simulink model "FOC_Motor_Control"  (R2020b)
settings: Solver=FixedStepAuto  StartTime=0.0  StopTime=10.0  FixedStep=Fixed_Step_Size  RelTol=1e-3
values from neighbouring files (symbols this model uses):
  Angle = 1.0    [Hall_FOC_Data.sldd]
  Angle_offset = 0.1985    [Hall_FOC_Data.sldd]
  atan_table = -1.5690511 -1.5690503 -1.5690495 -1.5690485 -1.5690477 -1.5690469 -1.569046 -1.5690452 -1.5690442 -1.5690434 -1.5690426 -1.5690417 -1.5690409 -1.5690399 -1.5690391 -1.5690383 -1.5690374 -1.5690365 -1.5690356 -1.5690348 -1.5690339 -1.569033 -1.5690322 -1.5690314 -1.5690304 -1.5690296 -1.5690287 -1.5690278 -1.5690269 -1.5690261 -1.5690252 -1.5690243 -1.5690234 -1.5690225 -1.5690217 -1.5690207 -1.569    [Hall_FOC_Data.sldd]
  Cosine_table = 1.0 0.99999529 0.99999058 0.99998587 0.99998116 0.99996704 0.99995291 0.99993885 0.99992472 0.99990118 0.99987763 0.99985409 0.9998306 0.99979764 0.99976468 0.99973178 0.99969882 0.99965644 0.99961412 0.99957174 0.99952942 0.99947762 0.99942589 0.99937415 0.99932235 0.9992612 0.99920005 0.99913889 0.99907768 0.99900717 0.99893659 0.99886602 0.99879545 0.99871546 0.99863547 0.99855554 0.99847555 0.    [Hall_FOC_Data.sldd]
  Dead_Com_Enable = 0.0    [Hall_FOC_Data.sldd]
  Dead_Time = 0.0    [Hall_FOC_Data.sldd]
  FF_Enable = 0.0    [Hall_FOC_Data.sldd]
  Flux = 0.0260812    [Hall_FOC_Data.sldd]
  FluxWeak_Enable = 0.0    [Hall_FOC_Data.sldd]
  FluxWeak_Idref_max = 0.0    [Hall_FOC_Data.sldd]
  FluxWeak_Idref_min = -200.0    [Hall_FOC_Data.sldd]
  FluxWeak_Ki = 50.0    [Hall_FOC_Data.sldd]
  FluxWeak_Kp = 1.2    [Hall_FOC_Data.sldd]
  HaLL_AngleShift = -0.25    [Hall_FOC_Data.sldd]
  HaLL_Sector1 = 5.236    [Hall_FOC_Data.sldd]
  HaLL_Sector2 = 1.0472    [Hall_FOC_Data.sldd]
  HaLL_Sector3 = 0.0    [Hall_FOC_Data.sldd]
  HaLL_Sector4 = 3.1415    [Hall_FOC_Data.sldd]
  HaLL_Sector5 = 4.1888    [Hall_FOC_Data.sldd]
  HaLL_Sector6 = 2.0944    [Hall_FOC_Data.sldd]
  HaLL_Timer_T = 1.0E-5    [Hall_FOC_Data.sldd]
  Harmonic_Com_Enable = 0.0    [Hall_FOC_Data.sldd]
  Harmonic_Id5th_Ki = 32.0    [Hall_FOC_Data.sldd]
  Harmonic_Id5th_Kp = 1.2    [Hall_FOC_Data.sldd]
  Harmonic_Id5th_Max = 60.0    [Hall_FOC_Data.sldd]
  Harmonic_Id5th_Min = -60.0    [Hall_FOC_Data.sldd]
  Harmonic_Id7th_Ki = 24.0    [Hall_FOC_Data.sldd]
  Harmonic_Id7th_Kp = 0.8    [Hall_FOC_Data.sldd]
  Harmonic_Id7th_Max = 60.0    [Hall_FOC_Data.sldd]
  Harmonic_Id7th_Min = -60.0    [Hall_FOC_Data.sldd]
  Harmonic_Iq5th_Ki = 32.0    [Hall_FOC_Data.sldd]
  Harmonic_Iq5th_Kp = 1.2    [Hall_FOC_Data.sldd]
  Harmonic_Iq5th_Max = 60.0    [Hall_FOC_Data.sldd]
  Harmonic_Iq5th_Min = -60.0    [Hall_FOC_Data.sldd]
  Harmonic_Iq7th_Ki = 24.0    [Hall_FOC_Data.sldd]
  Harmonic_Iq7th_Kp = 0.8    [Hall_FOC_Data.sldd]
  Harmonic_Iq7th_Max = 60.0    [Hall_FOC_Data.sldd]
  Harmonic_Iq7th_Min = -60.0    [Hall_FOC_Data.sldd]
  ID_Ki = 0.8    [Hall_FOC_Data.sldd]
  ID_Kp = 3.2    [Hall_FOC_Data.sldd]
  IQ_Ki = 0.32    [Hall_FOC_Data.sldd]
  IQ_Kp = 3.3    [Hall_FOC_Data.sldd]
  LADRC_b0 = 80000.0    [Hall_FOC_Data.sldd]
  LADRC_Omega_c = 80.0    [Hall_FOC_Data.sldd]
  Ld = 0.004    [Hall_FOC_Data.sldd]
  Lq = 0.0042    [Hall_FOC_Data.sldd]
  MTPA_id_table = 0.22889 0.23462678 0.23770036 0.2381243 0.23591207 0.23107713 0.2236329 0.21359272 0.20096992 0.18577772 0.16802935 0.14773798 0.12491672 0.099578641 0.071736768 0.041404068 0.0085934745 -0.026682133 -0.064409919 -0.10457709 -0.14717092 -0.1921787 -0.2395878 -0.28938559 -0.34155953 -0.39609709 -0.45298585 -0.51221335 -0.57376724 -0.63763517 -0.70380485 -0.77226412 -0.84300071 -0.91600245 -0.991257    [Hall_FOC_Data.sldd]
  MTPA_iq_table = -1.0417 -0.16083497 0.71926296 1.5985928 2.4771533 3.3549435 4.2319627 5.1082091 5.9836826 6.8583813 7.732305 8.6054525 9.4778223 10.349415 11.220228 12.090261 12.959513 13.827983 14.69567 15.562573 16.428694 17.294027 18.158575 19.022335 19.885307 20.747492 21.608887 22.469492 23.329306 24.188328 25.046556 25.903992 26.760633 27.616482 28.471533 29.325788 30.179247 31.031908 31.883772 32.734837 3    [Hall_FOC_Data.sldd]
  MTPA_Te_Max = 800.0    [Hall_FOC_Data.sldd]
  MTPA_Te_Min = 0.0    [Hall_FOC_Data.sldd]
  Over_modulation = 0.0    [Hall_FOC_Data.sldd]
  Pole_Pairs = 2.0    [Hall_FOC_Data.sldd]
  PWM_Frequency = 10000.0    [Hall_FOC_Data.sldd]
  R = 0.4    [Hall_FOC_Data.sldd]
  Sine_table = 0.0 0.0015339879 0.0030679768 0.0046019657 0.0061359555 0.0076698866 0.0092038177 0.010737749 0.012271681 0.013805497 0.015339312 0.016873131 0.018406944 0.019940587 0.021474229 0.023007872 0.024541514 0.026074925 0.027608337 0.029141748 0.03067516 0.032208283 0.033741407 0.035274528 0.036807653 0.038340431 0.039873205 0.04140598 0.042938754 0.04447113 0.046003502 0.047535874 0.049068246 0.0506001    [Hall_FOC_Data.sldd]
  Speed_Ki = 0.633    [Hall_FOC_Data.sldd]
  Speed_Kp = 0.0267    [Hall_FOC_Data.sldd]
  Speed_PI_OutputMax = 5.0    [Hall_FOC_Data.sldd]
  Speed_PI_OutputMin = -5.0    [Hall_FOC_Data.sldd]
  SpeedFilter_Fn = 0.2    [Hall_FOC_Data.sldd]
  TorqueMode = 0.0    [Hall_FOC_Data.sldd]
undefined symbols (not defined in the file or in its folder): DiscIntNeverNeededParam, inverter, magnitude, SVPWM
libraries: simulink x6, powerlib_extras x4, pid_lib x1
(part 5 of 5)

== system FOC_Motor_Control/Motor_Control/Motor_Control_Function/FOC_Control_100us/FOC/DT_Compensation/DT_Compensation/Subsystem/Subsystem2 ==
  Voltage : Inport
  Action Port : ActionPort  ActionPortLabel=elseif((u1 >1.570796)&(u1<=2.617993))
  Gain : Gain  Gain=-1
  Gain1 : Gain
  Gain2 : Gain  Gain=-1
  Mux1 : Mux  Inputs=3
  Out1 : Outport
  wires:
  Mux1/1 -> Out1/1
  Voltage/1 -> Gain2/1, Gain1/1, Gain/1
  Gain/1 -> Mux1/1
  Gain1/1 -> Mux1/2
  Gain2/1 -> Mux1/3

== system FOC_Motor_Control/Motor_Control/Motor_Control_Function/FOC_Control_100us/FOC/DT_Compensation/DT_Compensation/Subsystem/Subsystem3 ==
  Voltage : Inport
  Action Port : ActionPort  ActionPortLabel=elseif((u1 >2.617993)&(u1<=3.665191))
  Gain : Gain  Gain=-1
  Gain1 : Gain
  Gain2 : Gain
  Mux1 : Mux  Inputs=3
  Out1 : Outport
  wires:
  Mux1/1 -> Out1/1
  Voltage/1 -> Gain2/1, Gain1/1, Gain/1
  Gain/1 -> Mux1/1
  Gain1/1 -> Mux1/2
  Gain2/1 -> Mux1/3

== system FOC_Motor_Control/Motor_Control/Motor_Control_Function/FOC_Control_100us/FOC/DT_Compensation/DT_Compensation/Subsystem/Subsystem4 ==
  Voltage : Inport
  Action Port : ActionPort  ActionPortLabel=elseif((u1 >3.665191)&(u1<=4.7123889))
  Gain : Gain  Gain=-1
  Gain1 : Gain  Gain=-1
  Gain2 : Gain
  Mux1 : Mux  Inputs=3
  Out1 : Outport
  wires:
  Mux1/1 -> Out1/1
  Voltage/1 -> Gain2/1, Gain1/1, Gain/1
  Gain/1 -> Mux1/1
  Gain1/1 -> Mux1/2
  Gain2/1 -> Mux1/3

== system FOC_Motor_Control/Motor_Control/Motor_Control_Function/FOC_Control_100us/FOC/DT_Compensation/DT_Compensation/Subsystem/Subsystem5 ==
  Voltage : Inport
  Action Port : ActionPort  ActionPortLabel=elseif((u1 >4.7123889)&(u1<=5.75958))
  Gain : Gain
  Gain1 : Gain  Gain=-1
  Gain2 : Gain
  Mux1 : Mux  Inputs=3
  Out1 : Outport
  wires:
  Mux1/1 -> Out1/1
  Voltage/1 -> Gain2/1, Gain1/1, Gain/1
  Gain/1 -> Mux1/1
  Gain1/1 -> Mux1/2
  Gain2/1 -> Mux1/3

== system FOC_Motor_Control/Motor_Control/Motor_Control_Function/FOC_Control_100us/FOC/Har_Compensation/Har_Compensation/Idq5/LPF ==
  u : Inport
  Add : Sum  Inputs=+-
  Add1 : Sum
  Constant1 : Constant  Value=0.005  OutDataTypeStr=single
  Divide1 : Product  Inputs=**
  Unit Delay : UnitDelay  SampleTime=-1  HasFrameUpgradeWarning=on
  y : Outport
  wires:
  Constant1/1 -> Divide1/1
  u/1 -> Add/1
  Add/1 -> Divide1/2
  Divide1/1 -> Add1/1
  Unit Delay/1 -> Add/2, Add1/2
  Add1/1 -> Unit Delay/1, y/1

== system FOC_Motor_Control/Motor_Control/Motor_Control_Function/FOC_Control_100us/FOC/Har_Compensation/Har_Compensation/Idq5/LPF2 ==
  u : Inport
  Add : Sum  Inputs=+-
  Add1 : Sum
  Constant1 : Constant  Value=0.005  OutDataTypeStr=single
  Divide1 : Product  Inputs=**
  Unit Delay : UnitDelay  SampleTime=-1  HasFrameUpgradeWarning=on
  y : Outport
  wires:
  Constant1/1 -> Divide1/1
  u/1 -> Add/1
  Add/1 -> Divide1/2
  Divide1/1 -> Add1/1
  Unit Delay/1 -> Add/2, Add1/2
  Add1/1 -> Unit Delay/1, y/1

== system FOC_Motor_Control/Motor_Control/Motor_Control_Function/FOC_Control_100us/FOC/Har_Compensation/Har_Compensation/Idq5/Park1 ==
  Ialf : Inport
  Ibelt : Inport  Port=2
  Cos_theta : Inport  Port=3
  Sin_theta : Inport  Port=4
  Fcn2 : Fcn  Expr=u(1)*u(3)+u(2)*u(4)
  Fcn3 : Fcn  Expr=u(2)*u(3)-u(1)*u(4)
  Mux : Mux
  Id5 : Outport  VectorParamsAs1DForOutWhenUnconnected=off
  Iq5 : Outport  Port=2  VectorParamsAs1DForOutWhenUnconnected=off
  wires:
  Fcn3/1 -> Iq5/1
  Fcn2/1 -> Id5/1
  Mux/1 -> Fcn3/1, Fcn2/1
  Sin_theta/1 -> Mux/4
  Cos_theta/1 -> Mux/3
  Ibelt/1 -> Mux/2
  Ialf/1 -> Mux/1

== system FOC_Motor_Control/Motor_Control/Motor_Control_Function/FOC_Control_100us/FOC/Har_Compensation/Har_Compensation/Idq7/LPF ==
  u : Inport
  Add : Sum  Inputs=+-
  Add1 : Sum
  Constant1 : Constant  Value=0.005  OutDataTypeStr=single
  Divide1 : Product  Inputs=**
  Unit Delay : UnitDelay  SampleTime=-1  HasFrameUpgradeWarning=on
  y : Outport
  wires:
  Constant1/1 -> Divide1/1
  u/1 -> Add/1
  Add/1 -> Divide1/2
  Divide1/1 -> Add1/1
  Unit Delay/1 -> Add/2, Add1/2
  Add1/1 -> Unit Delay/1, y/1

== system FOC_Motor_Control/Motor_Control/Motor_Control_Function/FOC_Control_100us/FOC/Har_Compensation/Har_Compensation/Idq7/LPF2 ==
  u : Inport
  Add : Sum  Inputs=+-
  Add1 : Sum
  Constant1 : Constant  Value=0.005  OutDataTypeStr=single
  Divide1 : Product  Inputs=**
  Unit Delay : UnitDelay  SampleTime=-1  HasFrameUpgradeWarning=on
  y : Outport
  wires:
  Constant1/1 -> Divide1/1
  u/1 -> Add/1
  Add/1 -> Divide1/2
  Divide1/1 -> Add1/1
  Unit Delay/1 -> Add/2, Add1/2
  Add1/1 -> Unit Delay/1, y/1

== system FOC_Motor_Control/Motor_Control/Motor_Control_Function/FOC_Control_100us/FOC/Har_Compensation/Har_Compensation/Idq7/Park1 ==
  Ialf : Inport
  Ibelt : Inport  Port=2
  Cos_theta : Inport  Port=3
  Sin_theta : Inport  Port=4
  Fcn2 : Fcn  Expr=u(1)*u(3)+u(2)*u(4)
  Fcn3 : Fcn  Expr=u(2)*u(3)-u(1)*u(4)
  Mux : Mux
  Id7 : Outport  VectorParamsAs1DForOutWhenUnconnected=off
  Iq7 : Outport  Port=2  VectorParamsAs1DForOutWhenUnconnected=off
  wires:
  Ialf/1 -> Mux/1
  Ibelt/1 -> Mux/2
  Cos_theta/1 -> Mux/3
  Sin_theta/1 -> Mux/4
  Mux/1 -> Fcn2/1, Fcn3/1
  Fcn2/1 -> Id7/1
  Fcn3/1 -> Iq7/1

== system FOC_Motor_Control/Motor_Control/Motor_Control_Function/FOC_Control_100us/FOC/Har_Compensation/Har_Compensation/idq57_Controller/I-park ==
  Ud5 : Inport
  Uq5 : Inport  Port=2
  Cos_theta : Inport  Port=3
  Sin_theta : Inport  Port=4
  Fcn : Fcn  Expr=u(1)*u(3)-u(2)*u(4)
  Fcn1 : Fcn  Expr=u(1)*u(4)+u(2)*u(3)
  Mux1 : Mux
  Ualfa5 : Outport  VectorParamsAs1DForOutWhenUnconnected=off
  Ubelt5 : Outport  Port=2  VectorParamsAs1DForOutWhenUnconnected=off
  wires:
  Uq5/1 -> Mux1/2
  Ud5/1 -> Mux1/1
  Fcn1/1 -> Ubelt5/1
  Fcn/1 -> Ualfa5/1
  Mux1/1 -> Fcn1/1, Fcn/1
  Sin_theta/1 -> Mux1/4
  Cos_theta/1 -> Mux1/3

== system FOC_Motor_Control/Motor_Control/Motor_Control_Function/FOC_Control_100us/FOC/Har_Compensation/Har_Compensation/idq57_Controller/I-park1 ==
  Ud7 : Inport
  Uq7 : Inport  Port=2
  Cos_theta : Inport  Port=3
  Sin_theta : Inport  Port=4
  Fcn : Fcn  Expr=u(1)*u(3)-u(2)*u(4)
  Fcn1 : Fcn  Expr=u(1)*u(4)+u(2)*u(3)
  Mux1 : Mux
  Ualfa7 : Outport  VectorParamsAs1DForOutWhenUnconnected=off
  Ubelt7 : Outport  Port=2  VectorParamsAs1DForOutWhenUnconnected=off
  wires:
  Ud7/1 -> Mux1/1
  Fcn/1 -> Ualfa7/1
  Mux1/1 -> Fcn1/1, Fcn/1
  Fcn1/1 -> Ubelt7/1
  Uq7/1 -> Mux1/2
  Cos_theta/1 -> Mux1/3
  Sin_theta/1 -> Mux1/4

== system FOC_Motor_Control/Motor_Control/Motor_Control_Function/FOC_Control_100us/FOC/Har_Compensation/Har_Compensation/idq57_Controller/ID_5 ==
  Err : Inport
  Add : Sum
  Discrete-Time Integrator : DiscreteIntegrator  SampleTime=-1  ICPrevOutput=DiscIntNeverNeededParam  ICPrevScaledInput=DiscIntNeverNeededParam
  Ki : Constant  Value=Harmonic_Id5th_Ki  OutDataTypeStr=single
  Kp : Constant  Value=Harmonic_Id5th_Kp  OutDataTypeStr=single
  Product : Product
  Product1 : Product
  Saturation : Saturate  UpperLimit=Harmonic_Id5th_Max  LowerLimit=Harmonic_Id5th_Min
  PI_Out : Outport
  wires:
  Kp/1 -> Product/1
  Err/1 -> Product1/2, Product/2
  Product1/1 -> Discrete-Time Integrator/1
  Product/1 -> Add/1
  Add/1 -> Saturation/1
  Saturation/1 -> PI_Out/1
  Discrete-Time Integrator/1 -> Add/2
  Ki/1 -> Product1/1

== system FOC_Motor_Control/Motor_Control/Motor_Control_Function/FOC_Control_100us/FOC/Har_Compensation/Har_Compensation/idq57_Controller/ID_7 ==
  Err : Inport
  Add : Sum
  Discrete-Time Integrator : DiscreteIntegrator  SampleTime=-1  ICPrevOutput=DiscIntNeverNeededParam  ICPrevScaledInput=DiscIntNeverNeededParam
  Ki : Constant  Value=Harmonic_Id7th_Ki  OutDataTypeStr=single
  Kp : Constant  Value=Harmonic_Id7th_Kp  OutDataTypeStr=single
  Product : Product
  Product1 : Product
  Saturation : Saturate  UpperLimit=Harmonic_Id7th_Max  LowerLimit=Harmonic_Id7th_Min
  PI_Out : Outport
  wires:
  Kp/1 -> Product/1
  Err/1 -> Product1/2, Product/2
  Product1/1 -> Discrete-Time Integrator/1
  Product/1 -> Add/1
  Add/1 -> Saturation/1
  Saturation/1 -> PI_Out/1
  Discrete-Time Integrator/1 -> Add/2
  Ki/1 -> Product1/1

== system FOC_Motor_Control/Motor_Control/Motor_Control_Function/FOC_Control_100us/FOC/Har_Compensation/Har_Compensation/idq57_Controller/IQ_5 ==
  Err : Inport
  Add : Sum
  Discrete-Time Integrator : DiscreteIntegrator  SampleTime=-1  ICPrevOutput=DiscIntNeverNeededParam  ICPrevScaledInput=DiscIntNeverNeededParam
  Ki : Constant  Value=Harmonic_Iq5th_Ki  OutDataTypeStr=single
  Kp : Constant  Value=Harmonic_Iq5th_Kp  OutDataTypeStr=single
  Product : Product
  Product1 : Product
  Saturation : Saturate  UpperLimit=Harmonic_Iq5th_Max  LowerLimit=Harmonic_Iq5th_Min
  PI_Out : Outport
  wires:
  Kp/1 -> Product/1
  Err/1 -> Product1/2, Product/2
  Product1/1 -> Discrete-Time Integrator/1
  Product/1 -> Add/1
  Add/1 -> Saturation/1
  Saturation/1 -> PI_Out/1
  Discrete-Time Integrator/1 -> Add/2
  Ki/1 -> Product1/1

== system FOC_Motor_Control/Motor_Control/Motor_Control_Function/FOC_Control_100us/FOC/Har_Compensation/Har_Compensation/idq57_Controller/IQ_7 ==
  Err : Inport
  Add : Sum
  Discrete-Time Integrator : DiscreteIntegrator  SampleTime=-1  ICPrevOutput=DiscIntNeverNeededParam  ICPrevScaledInput=DiscIntNeverNeededParam
  Ki : Constant  Value=Harmonic_Iq7th_Ki  OutDataTypeStr=single
  Kp : Constant  Value=Harmonic_Iq7th_Kp  OutDataTypeStr=single
  Product : Product
  Product1 : Product
  Saturation : Saturate  UpperLimit=Harmonic_Iq7th_Max  LowerLimit=Harmonic_Iq7th_Min
  PI_Out : Outport
  wires:
  Kp/1 -> Product/1
  Err/1 -> Product1/2, Product/2
  Product1/1 -> Discrete-Time Integrator/1
  Product/1 -> Add/1
  Add/1 -> Saturation/1
  Saturation/1 -> PI_Out/1
  Discrete-Time Integrator/1 -> Add/2
  Ki/1 -> Product1/1

== system FOC_Motor_Control/Motor_Control/Motor_Control_Function/FOC_Control_100us/FOC/Har_Compensation/Har_Compensation/idq57_Controller/Subsystem1 ==
  note: id
  note: we
  Id7 : Inport
  We : Inport  Port=2
  Iq7 : Inport  Port=3
  Fcn : Fcn  Expr=-u(2)*Lq*u(3)+R*u(1)
  Fcn1 : Fcn  Expr=u(2)*Ld*u(1)+R*u(3)
  Mux1 : Mux  Inputs=3
  Udc7 : Outport  VectorParamsAs1DForOutWhenUnconnected=off
  Uqc7 : Outport  Port=2  VectorParamsAs1DForOutWhenUnconnected=off
  wires:
  Iq7/1 -> Mux1/3
  Mux1/1 -> Fcn/1, Fcn1/1
  Fcn/1 -> Udc7/1
  We/1 -> Mux1/2
  Fcn1/1 -> Uqc7/1
  Id7/1 -> Mux1/1

== system FOC_Motor_Control/Motor_Control/Motor_Control_Function/FOC_Control_100us/FOC/Har_Compensation/Har_Compensation/idq57_Controller/Subsystem2 ==
  note: we
  note: id
  Id5 : Inport
  We : Inport  Port=2
  Iq5 : Inport  Port=3
  Fcn : Fcn  Expr=u(2)*Lq*u(3)+R*u(1)
  Fcn1 : Fcn  Expr=-u(2)*Ld*u(1)+R*u(3)
  Mux1 : Mux  Inputs=3
  Udc5 : Outport  VectorParamsAs1DForOutWhenUnconnected=off
  Uqc5 : Outport  Port=2  VectorParamsAs1DForOutWhenUnconnected=off
  wires:
  Id5/1 -> Mux1/1
  Fcn1/1 -> Uqc5/1
  We/1 -> Mux1/2
  Fcn/1 -> Udc5/1
  Mux1/1 -> Fcn/1, Fcn1/1
  Iq5/1 -> Mux1/3

== system FOC_Motor_Control/Motor_Control/Motor_Control_Function/FOC_Control_100us/FOC/DT_Compensation/DT_Compensation/IsTheta_Cal/Angle_calibration/If Action Subsystem1 ==
  Angle_input : Inport
  Action Port : ActionPort  ActionPortLabel=else
  Out1 : Outport
  wires:
  Angle_input/1 -> Out1/1

== system FOC_Motor_Control/Motor_Control/Motor_Control_Function/FOC_Control_100us/FOC/DT_Compensation/DT_Compensation/IsTheta_Cal/Angle_calibration/If Action Subsystem2 ==
  In1 : Inport
  Action Port : ActionPort  ActionPortLabel=if(u1 > 6.283185307)
  2pi : Constant  Value=2*pi  OutDataTypeStr=single
  Subtract1 : Sum  Inputs=+-
  Out1 : Outport
  wires:
  In1/1 -> Subtract1/1
  Subtract1/1 -> Out1/1
  2pi/1 -> Subtract1/2

== system FOC_Motor_Control/Motor_Control/Motor_Control_Function/FOC_Control_100us/FOC/DT_Compensation/DT_Compensation/IsTheta_Cal/atan/If Action Subsystem10 ==
  A_iq : Inport
  B_id : Inport  Port=2
  Action Port : ActionPort  ActionPortLabel=if((u1<0)&(u2<0))
  1-D Lookup Table4 : Lookup_n-D  NumberOfTableDimensions=1  LookupTableObject=''  BreakpointsForDimension1=single(linspace(-573,573,length(atan_table)));  BreakpointsForDimension1FirstPoint=10  BreakpointsForDimension2FirstPoint=10  BreakpointsForDimension1Spacing=12  BreakpointsForDimension2Spacing=12  IndexSearchMethod=Evenly spaced points  Table=atan_table  InterpMethod=Flat  DiagnosticForOutOfRangeInput=Error  InternalRulePriority=Speed  RndMeth=Simplest  InputSameDT=on
  Add : Sum  Inputs=+-
  Constant : Constant  Value=pi  OutDataTypeStr=single
  Divide : Product  Inputs=*/
  Saturation : Saturate  UpperLimit=572  LowerLimit=-572
  Scope : Scope
  IsTheta : Outport
  wires:
  Add/1 -> IsTheta/1
  Saturation/1 -> Scope/1, 1-D Lookup Table4/1
  A_iq/1 -> Divide/1
  Constant/1 -> Add/2
  Divide/1 -> Saturation/1
  B_id/1 -> Divide/2
  1-D Lookup Table4/1 -> Add/1

== system FOC_Motor_Control/Motor_Control/Motor_Control_Function/FOC_Control_100us/FOC/DT_Compensation/DT_Compensation/IsTheta_Cal/atan/If Action Subsystem11 ==
  Action Port : ActionPort  ActionPortLabel=if((u1>0)&(u2==0))
  Constant : Constant  Value=pi/2  OutDataTypeStr=single
  IsTheta : Outport
  wires:
  Constant/1 -> IsTheta/1

== system FOC_Motor_Control/Motor_Control/Motor_Control_Function/FOC_Control_100us/FOC/DT_Compensation/DT_Compensation/IsTheta_Cal/atan/If Action Subsystem12 ==
  Action Port : ActionPort  ActionPortLabel=if((u1<0)&(u2==0))
  Constant : Constant  Value=-pi/2  OutDataTypeStr=single
  IsTheta : Outport
  wires:
  Constant/1 -> IsTheta/1

== system FOC_Motor_Control/Motor_Control/Motor_Control_Function/FOC_Control_100us/FOC/DT_Compensation/DT_Compensation/IsTheta_Cal/atan/If Action Subsystem8 ==
  A_iq : Inport
  B_id : Inport  Port=2
  Action Port : ActionPort  ActionPortLabel=if((u1 >0))
  1-D Lookup Table4 : Lookup_n-D  NumberOfTableDimensions=1  LookupTableObject=''  BreakpointsForDimension1=single(linspace(-573,573,length(atan_table)));  BreakpointsForDimension1FirstPoint=10  BreakpointsForDimension2FirstPoint=10  BreakpointsForDimension1Spacing=12  BreakpointsForDimension2Spacing=12  IndexSearchMethod=Evenly spaced points  Table=atan_table  InterpMethod=Flat  DiagnosticForOutOfRangeInput=Error  InternalRulePriority=Speed  RndMeth=Simplest  InputSameDT=on
  Divide : Product  Inputs=*/
  Saturation : Saturate  UpperLimit=572  LowerLimit=-572
  Scope : Scope  NumInputPorts=2
  IsTheta : Outport
  wires:
  Divide/1 -> Saturation/1
  A_iq/1 -> Divide/1
  B_id/1 -> Divide/2
  Saturation/1 -> Scope/1, 1-D Lookup Table4/1
  1-D Lookup Table4/1 -> Scope/2, IsTheta/1

== system FOC_Motor_Control/Motor_Control/Motor_Control_Function/FOC_Control_100us/FOC/DT_Compensation/DT_Compensation/IsTheta_Cal/atan/If Action Subsystem9 ==
  A_iq : Inport
  B_id : Inport  Port=2
  Action Port : ActionPort  ActionPortLabel=if((u1>=0)&(u2<0))
  1-D Lookup Table4 : Lookup_n-D  NumberOfTableDimensions=1  LookupTableObject=''  BreakpointsForDimension1=single(linspace(-573,573,length(atan_table)));  BreakpointsForDimension1FirstPoint=10  BreakpointsForDimension2FirstPoint=10  BreakpointsForDimension1Spacing=12  BreakpointsForDimension2Spacing=12  IndexSearchMethod=Evenly spaced points  Table=atan_table  InterpMethod=Flat  DiagnosticForOutOfRangeInput=Error  InternalRulePriority=Speed  RndMeth=Simplest  InputSameDT=on
  Add : Sum
  Constant : Constant  Value=pi  OutDataTypeStr=single
  Divide : Product  Inputs=*/
  Saturation : Saturate  UpperLimit=572  LowerLimit=-572
  Scope : Scope  NumInputPorts=3
  IsTheta : Outport
  wires:
  B_id/1 -> Divide/2
  A_iq/1 -> Divide/1
  Add/1 -> Scope/3, IsTheta/1
  Constant/1 -> Add/2
  Saturation/1 -> Scope/1, 1-D Lookup Table4/1
  Divide/1 -> Saturation/1
  1-D Lookup Table4/1 -> Scope/2, Add/1
